simulink model "ThirdSimulinkQUstion"  (R2020b)
settings: Solver=VariableStepAuto  StartTime=0.0  StopTime=10.0  RelTol=1e-3
libraries: simulink x1
settings Model: Creator=parke  LastModifiedBy=parke

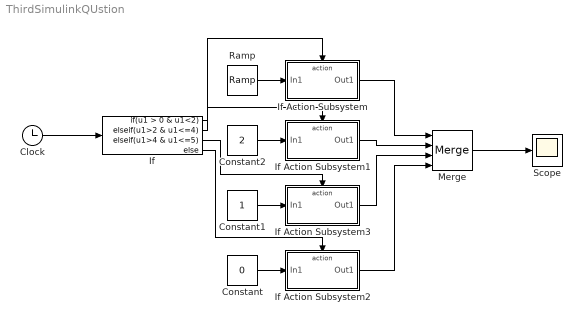
== system ThirdSimulinkQUstion ==
  Clock : Clock
  Constant : Constant  Value=0
  Constant1 : Constant
  Constant2 : Constant  Value=2
  If : If  IfExpression=u1 > 0 & u1<2  ElseIfExpressions=u1>2 & u1<=4, u1>4 & u1<=5
  If Action Subsystem : Subsystem  TreatAsAtomicUnit=on
  If Action Subsystem1 : Subsystem  TreatAsAtomicUnit=on
  If Action Subsystem2 : Subsystem  TreatAsAtomicUnit=on
  If Action Subsystem3 : Subsystem  TreatAsAtomicUnit=on
  Merge : Merge  Inputs=4
  Ramp : simulink/Sources/Ramp  slope=1  start=0  InitialOutput=0
  Scope : Scope
  wires:
  Clock/1 -> If/1
  If/1 -> If Action Subsystem/Action
  If/2 -> If Action Subsystem1/Action
  If/4 -> If Action Subsystem2/Action
  If/3 -> If Action Subsystem3/Action
  Constant/1 -> If Action Subsystem2/1(In1)
  Constant1/1 -> If Action Subsystem3/1(In1)
  Constant2/1 -> If Action Subsystem1/1(In1)
  Ramp/1 -> If Action Subsystem/1(In1)
  If Action Subsystem/1(Out1) -> Merge/1
  If Action Subsystem1/1(Out1) -> Merge/2
  If Action Subsystem3/1(Out1) -> Merge/3
  If Action Subsystem2/1(Out1) -> Merge/4
  Merge/1 -> Scope/1

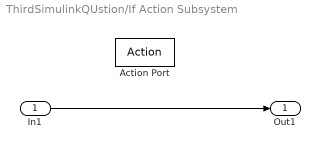
== system ThirdSimulinkQUstion/If Action Subsystem ==
  In1 : Inport
  Action Port : ActionPort  ActionPortLabel=if(u1 > 0 & u1<2)
  Out1 : Outport
  wires:
  In1/1 -> Out1/1

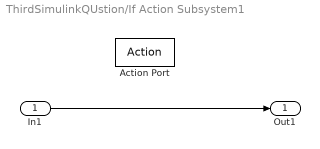
== system ThirdSimulinkQUstion/If Action Subsystem1 ==
  In1 : Inport
  Action Port : ActionPort  ActionPortLabel=elseif(u1>2 & u1<=4)
  Out1 : Outport
  wires:
  In1/1 -> Out1/1

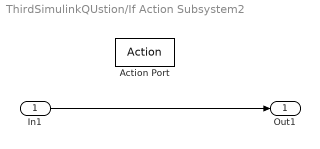
== system ThirdSimulinkQUstion/If Action Subsystem2 ==
  In1 : Inport
  Action Port : ActionPort  ActionPortLabel=else
  Out1 : Outport
  wires:
  In1/1 -> Out1/1

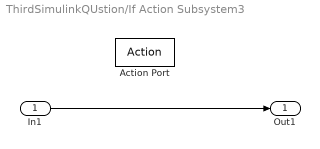
== system ThirdSimulinkQUstion/If Action Subsystem3 ==
  In1 : Inport
  Action Port : ActionPort  ActionPortLabel=elseif( u1>4 & u1<=5)
  Out1 : Outport
  wires:
  In1/1 -> Out1/1
